simulink model "siude"  (Simulink 8.5)
settings: Solver=ode4  StartTime=0.0  StopTime=tstop  FixedStep=tstep  RelTol=1e-3
values from neighbouring files (symbols this model uses):
  const = -6/(bpnom * delt^3)    (= 0.279524420401)    [dataude.m]
settings Model: Creator=Dr SE Talole  LastModifiedBy=Vish
settings OptimizationCC: InitFltsAndDblsToZero=on
settings DebuggingCC: SaveWithParameterizedLinksMsg=none  SignalResolutionControl=TryResolveAllWithWarning  SolverPrmCheckMsg=warning  MultiTaskDSMMsg=warning  MultiTaskCondExecSysMsg=none  FcnCallInpInsideContextMsg=UseLocalSettings
settings GRTTargetCC: TargetFcnLib=ansi_tfl_tmw.mat

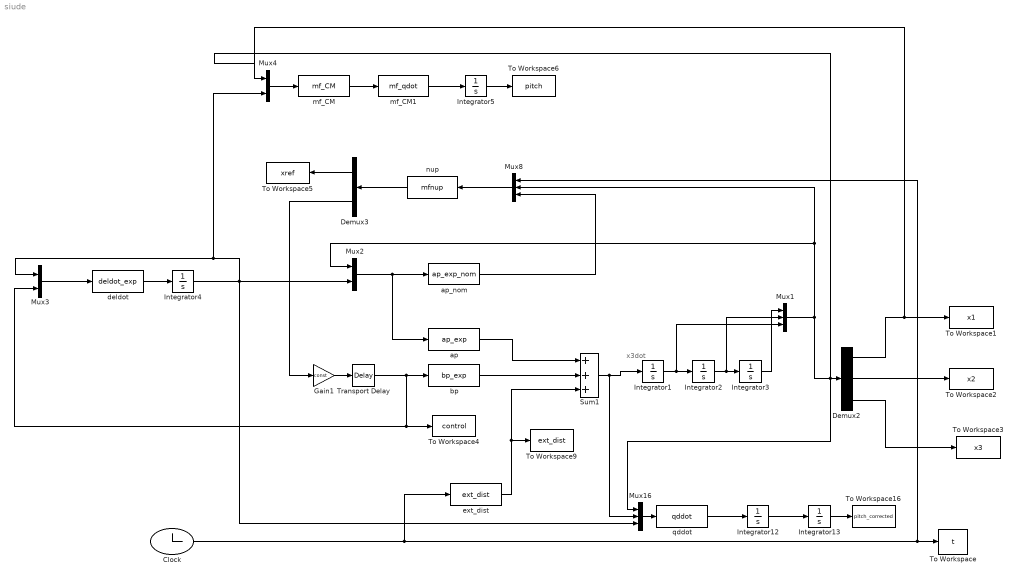
== system siude ==
  note: x3dot
  Clock : Clock
  Demux2 : Demux  Outputs=3
  Demux3 : Demux  Outputs=2
  Gain1 : Gain  Gain=const
  Integrator{1..5,12..13} (7 alike) : Integrator
  Mux1 : Mux  Inputs=3
  Mux16 : Mux  Inputs=3
  Mux2 : Mux  Inputs=2
  Mux3 : Mux  Inputs=2
  Mux4 : Mux  Inputs=2
  Mux8 : Mux  Inputs=3
  Sum1 : Sum  Inputs=+++
  To Workspace : ToWorkspace  VariableName=t  SampleTime=-1
  To Workspace1 : ToWorkspace  VariableName=x1  SampleTime=-1
  To Workspace16 : ToWorkspace  VariableName=pitch_corrected  SampleTime=-1
  To Workspace2 : ToWorkspace  VariableName=x2  SampleTime=-1
  To Workspace3 : ToWorkspace  VariableName=x3  SampleTime=-1
  To Workspace4 : ToWorkspace  VariableName=control  SampleTime=-1
  To Workspace5 : ToWorkspace  VariableName=xref  SampleTime=-1
  To Workspace6 : ToWorkspace  VariableName=pitch  SampleTime=-1
  To Workspace9 : ToWorkspace  VariableName=ext_dist  SampleTime=-1
  Transport Delay : TransportDelay  DelayTime=0
  ap : MATLABFcn  MATLABFcn=ap_exp  OutputDimensions=1
  "ap_nom " : MATLABFcn  MATLABFcn=ap_exp_nom  OutputDimensions=1
  bp : MATLABFcn  MATLABFcn=bp_exp  OutputDimensions=1
  deldot : MATLABFcn  MATLABFcn=deldot_exp  OutputDimensions=1
  "ext_dist " : MATLABFcn  MATLABFcn=ext_dist  OutputDimensions=1
  mf_CM : MATLABFcn  MATLABFcn=mf_CM  OutputDimensions=1
  mf_CM1 : MATLABFcn  MATLABFcn=mf_qdot  OutputDimensions=1
  nup : MATLABFcn  MATLABFcn=mfnup  OutputDimensions=2
  qddot : MATLABFcn  MATLABFcn=qddot  OutputDimensions=1
  wires:
  Integrator3/1 -> Mux1/1
  Integrator2/1 -> Mux1/2, Integrator3/1
  Integrator1/1 -> Mux1/3, Integrator2/1
  Demux2/2 -> To Workspace2/1
  ap/1 -> Sum1/1
  Mux2/1 -> ap/1, "ap_nom "/1
  Mux3/1 -> deldot/1
  deldot/1 -> Integrator4/1
  Integrator4/1 -> Mux4/2, Mux3/1, Mux16/3, Mux2/2
  Demux2/3 -> To Workspace3/1
  Sum1/1 -> Mux16/2, Integrator1/1
  Mux1/1 -> Mux8/2, Mux2/1, Mux16/1, Demux2/1
  Demux2/1 -> Mux4/1, To Workspace1/1
  Transport Delay/1 -> bp/1, Mux3/2, To Workspace4/1
  bp/1 -> Sum1/2
  Clock/1 -> Mux8/1, To Workspace/1, "ext_dist "/1
  "ext_dist "/1 -> Sum1/3, To Workspace9/1
  nup/1 -> Demux3/1
  Mux8/1 -> nup/1
  Demux3/2 -> Gain1/1
  Demux3/1 -> To Workspace5/1
  "ap_nom "/1 -> Mux8/3
  Mux4/1 -> mf_CM/1
  mf_CM/1 -> mf_CM1/1
  mf_CM1/1 -> Integrator5/1
  Integrator5/1 -> To Workspace6/1
  Gain1/1 -> Transport Delay/1
  Mux16/1 -> qddot/1
  qddot/1 -> Integrator12/1
  Integrator12/1 -> Integrator13/1
  Integrator13/1 -> To Workspace16/1
